simulink model "sm_car_testrig_susp_dwa_hp"  (R2025b)
settings: Solver=ode23t  StartTime=0.0  StopTime=1e-9  RelTol=1e-3  EnableMultiTasking=on
PostLoadFcn:
  | sm_car_load_vehicle_data(bdroot,'016');
undefined symbols (not defined in the file): Init, LAf, LAr, UAf, UAr, Vehicle, X, Y, Z
libraries: sm_lib x102, nesl_utility x67, Suspension_Utilities x8, Linkage_Arms x6, Linkage_DW_A x4, fl_lib x4, Linkage_Shock x2, Linkage_Uprights x2
(part 1 of 4)
Description:
  | Hardpoint Testrig for Double-Wishbone, Design A
  | 
  | Copyright 2018-2025 The MathWorks, Inc.
settings Model: Creator=smiller  LastModifiedBy=smiller
settings SolverCC: AlgebraicLoopSolver=TrustRegion
settings DataIOCC: LimitDataPoints=on  ReturnWorkspaceOutputs=off
settings OptimizationCC: ReuseModelBlockBuffer=off  LifeSpan=inf
settings DebuggingCC: UnconnectedInputMsg=warning  UnconnectedOutputMsg=warning  UnconnectedLineMsg=warning  AllowSymbolicDim=off  SFUnexpectedBacktrackingDiag=warning  SFNoUnconditionalDefaultTransitionDiag=warning  SFExecutionAtInitializationDiag=none  ArithmeticOperatorsInVariantConditions=warning
settings ModelReferenceCC: EnableRefExpFcnMdlSchedulingChecks=on
settings SFSimCC: SimUseLocalCustomCode=off  CustomCodeUndefinedFunction=UseInterfaceOnly
settings RTWCC: RTWUseLocalCustomCode=off  GPUComputeCapability=3.5  DLArmComputeVersion=19.05
settings CodeAppCC: StateflowObjectComments=on
settings GRTTargetCC: TargetLangStandard=C89/C90 (ANSI)
settings ConfigComp: CovMetricSettings=dw  CovSaveCumulativeToWorkspaceVar=on  CovSaveSingleToWorkspaceVar=on  CovExternalEMLEnable=off  CovSFcnEnable=off
settings SimscapeCC: SimscapeNominalValues="[{\"value\":\"10\",\"unit\":\"V\"},{\"value\":\"1\",\"unit\":\"A\"},{\"value\":\"10\",\"unit\":\"N*m\"},{\"value\":\"10\",\"unit\":\"bar\"},{\"value\":\"100\",\"unit\":\"kJ/kg\"},{\"value\":\"1\",\"unit\":\"kW\"},{\"value\":\"300\",\"unit\":\"K\"},{\"value\":\"100\",\"unit\":\"cm^3/s\"},{\"value\":\"1\",\"unit\":\"kN\"},{\"value\":\"1\",\"unit\":\"g/cm^3\"},{\"value\":\"1\",\"unit\":\"l\"},{\"value\":\"1\",\"unit\":\"cm^2\"},{\"value\":\"60\",\"unit\":\"Hz\"}]"  SimscapeLogType=all  SimscapeLogDataHistory=10000.0
settings ConfigurationSet: Description=SimMechanics 2G
settings ExplorerConfigSet: InternalSimMechanicsExplorerSettings="<ExplorerConfiguration><canonicalview>default</canonicalview><AnimationSetting><BasePlaybackSpeed>1.0</BasePlaybackSpeed><PlaybackSpeedFactor>1.0</PlaybackSpeedFactor></AnimationSetting><TilePanel><TileInfo><Tiles Columns=\"1\" Count=\"2\" Rows=\"2\"><Column Weight=\"1\"/><Row Weight=\"0.4725\"/><Row Weight=\"0.5275\"/><Tile Height=\"1\" Width=\"1\" X=\"0\" Y=\"0\"/><Tile Height=\"1\" Width=\"1\" X=\"0\" Y=\"1\"/></Tiles></TileInfo><SceneInfo><SceneViewer><BGColor><R>1</R><G>1</G><B>1</B></BGColor><Camera><DoPerspective>off</DoPerspective><Position><X>0.0507207717361932015</X><Y>0.00200032852270663059</Y><Z>1.76122408385226614</Z></Position><Center><X>0.0507207717361932015</X><Y>0.00200032852270663059</Y><Z>0.418399934818852515</Z></Center><Up><X>0.999884344159155392</X><Y>0.015208494515101291</Y><Z>0</Z></Up><ViewLimDist>1</ViewLimDist><YLim>0.36770677816381625</YLim><XLim>1.19032707650096015</XLim></Camera></SceneViewer><SceneViewer><BGColor><R>1</R><G>1</G><B>1</B></BGColor><Camera><DoPerspective>off</DoPerspective><Position><X>-1.166386773956821</X><Y>3.31266427622267656e-08</Y><Z>0.418399978770330305</Z></Position><Center><X>0.0499999423256101139</X><Y>3.31266427622267656e-08</Y><Z>0.418399978770330305</Z></Center><Up><X>0</X><Y>0</Y><Z>1</Z></Up><ViewLimDist>1</ViewLimDist><YLim>0.416223000884056116</YLim><XLim>1.20586269840369886</XLim></Camera></SceneViewer></SceneInfo></TilePanel><MechEditorPanel><Cameras/><GfxPanelCameraMap/><VideoCreator><PlaybackSpeedRatio>1.0</PlaybackSpeedRatio><FrameRate>30</FrameRate><VideoFormat>Motion JPEG AVI</VideoFormat><FrameSize>auto</FrameSize></VideoCreator></MechEditorPanel></ExplorerConfiguration>"

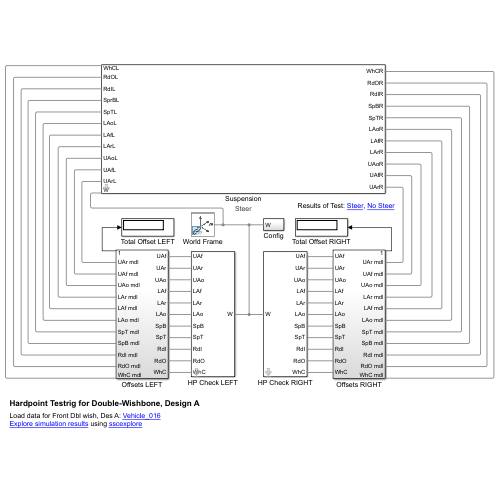
[thumbnail: Simulink's stored preview of the top-level diagram]
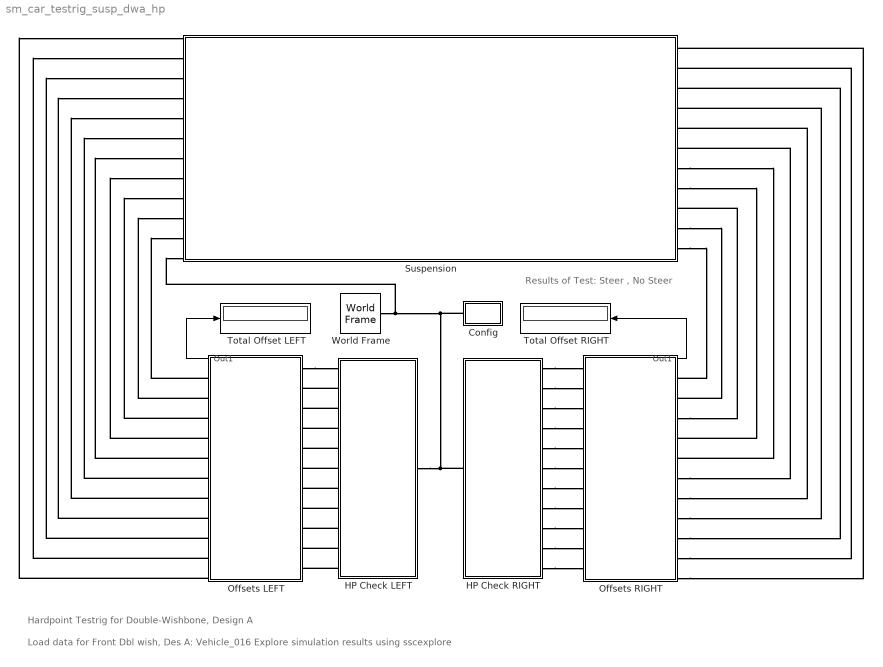
== system sm_car_testrig_susp_dwa_hp ==
  note: Results of Test: Steer , No Steer
  note: Hardpoint Testrig for Double-Wishbone, Design A
  note: Load data for Front Dbl wish, Des A: Vehicle_016
      | Explore simulation results using sscexplore
  Config : Subsystem
  HP Check LEFT : Subsystem  mask{Linkage=Vehicle.Chassis.SuspA1.Linkage, popup_leftRight=Left, rad_vis_sph=5e-2, clr_vis_sph=[0.4 0.4 1.0], opc_vis_sph=0.4, size_frm_vis=20, clr_frm_vis=[0.4 0.4 1.0], opc_frm_vis=0.5}
      mask prompts: Linkage "Linkage Parameters"; popup_leftRight "Left/Right"; rad_vis_sph "Sphere Radius (m)"; clr_vis_sph "Sphere Color [RGB]"; opc_vis_sph "Sphere Opacity (0-1)"; size_frm_vis "Frame Size (pixels)"; clr_frm_vis "Frame Color [RGB]"; opc_frm_vis "Frame Opacity (0-1)"
      mask init:
      | if(popup_leftRight==1)
      |     rhs_hp = [1 1 1];
      | elseif (popup_leftRight==2)
      |     rhs_hp = [1 -1 1];
      | end
      mask TypeOptions popup_leftRight: Left | Right
  HP Check RIGHT : Subsystem  mask{Linkage=Vehicle.Chassis.SuspA1.Linkage, popup_leftRight=Right, rad_vis_sph=5e-2, clr_vis_sph=[0.4 0.4 1.0], opc_vis_sph=0.4, size_frm_vis=20, clr_frm_vis=[0.4 0.4 1.0], opc_frm_vis=0.5}
      mask prompts: Linkage "Linkage Parameters"; popup_leftRight "Left/Right"; rad_vis_sph "Sphere Radius (m)"; clr_vis_sph "Sphere Color [RGB]"; opc_vis_sph "Sphere Opacity (0-1)"; size_frm_vis "Frame Size (pixels)"; clr_frm_vis "Frame Color [RGB]"; opc_frm_vis "Frame Opacity (0-1)"
      mask init:
      | if(popup_leftRight==1)
      |     rhs_hp = [1 1 1];
      | elseif (popup_leftRight==2)
      |     rhs_hp = [1 -1 1];
      | end
      mask TypeOptions popup_leftRight: Left | Right
  Offsets LEFT : Subsystem
  Offsets RIGHT : Subsystem
  Suspension : Subsystem  mask{popup_steer=Steer, Linkage=Vehicle.Chassis.SuspA1.Linkage}
      mask prompts: popup_steer "Steer (On/Off)"; Linkage "Linkage Parameters"
      mask init:
      | if (popup_steer == 1)
      |     set_param([gcb '/Track Rod LEFT'],'OverrideUsingVariant','Steer');
      |     set_param([gcb '/LA Upright LEFT'],'OverrideUsingVariant','Steer');
      |     set_param([gcb '/Track Rod RIGHT'],'OverrideUsingVariant','Steer');
      |     set_param([gcb '/LA Upright RIGHT'],'OverrideUsingVariant','Steer');
      | elseif (popup_steer == 2)
      |     set_param([gcb '/Track Rod LEFT'],'OverrideUsingVariant','No_Steer');
      |     set_param([gcb '/LA Upright LEFT'],'OverrideUsingVariant','No_Steer');
      |     set_param([gcb '/Track Rod RIGHT'],'OverrideUsingVariant','No_Steer');
      |     set_param([gcb '/LA Upright RIGHT'],'OverrideUsingVariant','No_Steer');
      | end
      settings: AttributesFormatString=%<popup_steer>
      mask TypeOptions popup_steer: Steer | No Steer
  Total Offset LEFT : Display
  Total Offset RIGHT : Display
  World Frame : sm_lib/Frames and Transforms/World Frame
  wires:
  Offsets LEFT/1(Out1) -> Total Offset LEFT/1
  Offsets RIGHT/1(Out1) -> Total Offset RIGHT/1
  connections:
  Offsets LEFT/LConn1 -- HP Check LEFT/RConn1
  HP Check LEFT/RConn2 -- Offsets LEFT/LConn2
  HP Check LEFT/RConn3 -- Offsets LEFT/LConn3
  HP Check LEFT/RConn4 -- Offsets LEFT/LConn4
  HP Check LEFT/RConn5 -- Offsets LEFT/LConn5
  HP Check LEFT/RConn6 -- Offsets LEFT/LConn6
  HP Check LEFT/RConn7 -- Offsets LEFT/LConn7
  HP Check LEFT/RConn8 -- Offsets LEFT/LConn8
  HP Check LEFT/RConn9 -- Offsets LEFT/LConn9
  HP Check LEFT/RConn10 -- Offsets LEFT/LConn10
  HP Check LEFT/RConn11 -- Offsets LEFT/LConn11
  HP Check RIGHT/RConn1 -- Offsets RIGHT/LConn1
  HP Check RIGHT/RConn2 -- Offsets RIGHT/LConn2
  HP Check RIGHT/RConn3 -- Offsets RIGHT/LConn3
  HP Check RIGHT/RConn4 -- Offsets RIGHT/LConn4
  HP Check RIGHT/RConn5 -- Offsets RIGHT/LConn5
  HP Check RIGHT/RConn6 -- Offsets RIGHT/LConn6
  HP Check RIGHT/RConn7 -- Offsets RIGHT/LConn7
  HP Check RIGHT/RConn8 -- Offsets RIGHT/LConn8
  HP Check RIGHT/RConn9 -- Offsets RIGHT/LConn9
  HP Check RIGHT/RConn10 -- Offsets RIGHT/LConn10
  HP Check RIGHT/RConn11 -- Offsets RIGHT/LConn11
  World Frame/RConn1 -- HP Check RIGHT/LConn1 -- HP Check LEFT/LConn1 -- Config/LConn1 -- Suspension/LConn12
  Offsets LEFT/RConn1 -- Suspension/LConn11
  Suspension/RConn11 -- Offsets RIGHT/RConn1
  Offsets LEFT/RConn2 -- Suspension/LConn10
  Suspension/RConn10 -- Offsets RIGHT/RConn2
  Offsets LEFT/RConn3 -- Suspension/LConn9
  Offsets RIGHT/RConn3 -- Suspension/RConn9
  Offsets LEFT/RConn4 -- Suspension/LConn8
  Suspension/RConn8 -- Offsets RIGHT/RConn4
  Offsets LEFT/RConn5 -- Suspension/LConn7
  Suspension/RConn7 -- Offsets RIGHT/RConn5
  Offsets LEFT/RConn6 -- Suspension/LConn6
  Offsets RIGHT/RConn6 -- Suspension/RConn6
  Offsets LEFT/RConn7 -- Suspension/LConn5
  Offsets RIGHT/RConn7 -- Suspension/RConn5
  Offsets LEFT/RConn8 -- Suspension/LConn4
  Offsets RIGHT/RConn8 -- Suspension/RConn4
  Offsets LEFT/RConn9 -- Suspension/LConn3
  Offsets RIGHT/RConn9 -- Suspension/RConn3
  Offsets LEFT/RConn10 -- Suspension/LConn2
  Offsets RIGHT/RConn10 -- Suspension/RConn2
  Offsets LEFT/RConn11 -- Suspension/LConn1
  Offsets RIGHT/RConn11 -- Suspension/RConn1

== system sm_car_testrig_susp_dwa_hp/Config ==
  Mechanism Configuration : sm_lib/Utilities/Mechanism Configuration  UniformGravity=Constant  GravityVector=[0 0 -9.80665]  GravityVectorUnits=m/s^2  LinearizationDelta=0.001  JointModeTransitionNonlinearIterations=2
  Solver Configuration : nesl_utility/Solver Configuration  PhysicalDomain=network_engine_domain  SubClassName=solver  LeftPortType=input  RightPortType=generic  Tones=[]  Harmonics=[]  SimulateNoise=off  Profile=off  UseLocalSampling=off  EnableSwitchedLinearOptims=on  FrequencyDomain=off  UseCCode=off  RelTol=0.001  AbsTol=1e-06  MinStep=1e-09  ToWorkspace=off  RevertToSquareIcSolve=off  NumHomotopyIterations=100  PhasorMode=off  PhasorModeNumHarmonics=1  ConsistencySolver=NEWTON_FTOL  IndexReductionMethod=DerivativeReplacement  DoDC=off  ResidualTolerance=1e-09  ConsistencyTolSource=GLOBAL  ConsistencyAbsTol=0.001  ConsistencyRelTol=0.001  ConsistencyTolFactor=0.001  UseLocalSolver=off  LocalSolverChoice=NE_BACKWARD_EULER_ADVANCER  ResolveIndetEquations=on  FunctionEvalNumThread=1  LocalSolverSampleTime=0.001  DoFixedCost=off  MaxNonlinIter=3  MaxModeIter=2  ComputeImpulses=off  ImpulseIterations=2  LinearAlgebra=Sparse  LinearAlgebraNumThread=0  EquationFormulation=NE_TIME_EF  DelaysMemoryBudget=1024  AutomaticFiltering=on  FilteringTimeConstant=0.001  PartitionStorageMethod=AS_NEEDED  PartitionMemoryBudget=1024  PartitionMethod=FAST  MultibodyUseLocalSolver=off  MultibodyLocalSolverChoice=ODE1  MultibodyLocalSolverSampleTime=0.001
  W : PMIOPort  Side=Left
  connections:
  Mechanism Configuration/RConn1 -- Solver Configuration/RConn1 -- W/RConn1

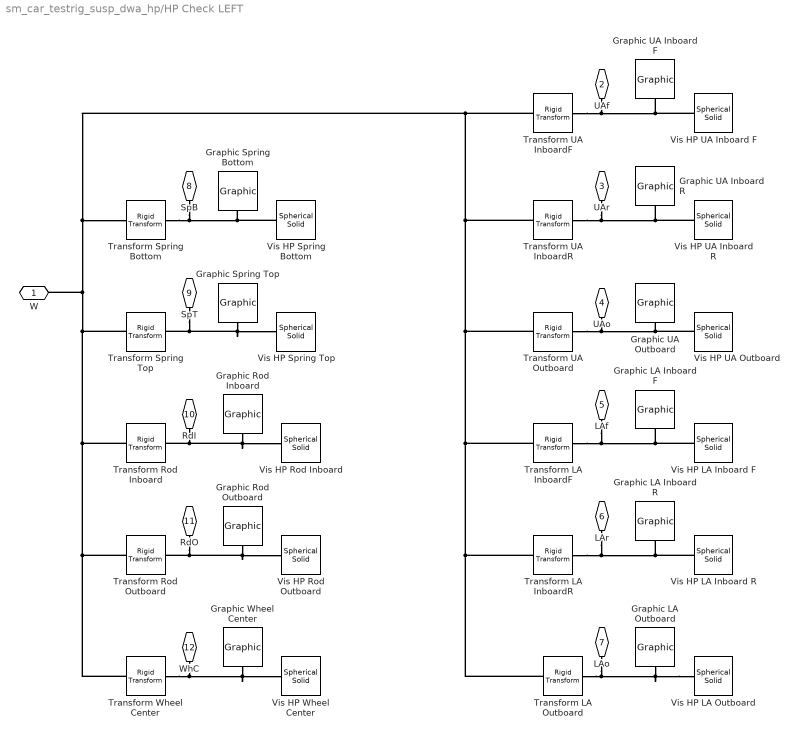
== system sm_car_testrig_susp_dwa_hp/HP Check LEFT ==
  Graphic LA Inboard F : sm_lib/Body Elements/Graphic  GraphicType=Marker  MarkerShape=Frame  MarkerSize=size_frm_vis  GraphicVisPropType=SimpleVisualProperties  GraphicDiffuseColor=clr_frm_vis  GraphicOpacity=opc_frm_vis  GraphicSpecularColor=[0.5 0.5 0.5 1.0]  GraphicAmbientColor=[0.15 0.15 0.15 1.0]  GraphicEmissiveColor=[0.0 0.0 0.0 1.0]  GraphicShininess=75
  Graphic LA Inboard R : sm_lib/Body Elements/Graphic  GraphicType=Marker  MarkerShape=Frame  MarkerSize=size_frm_vis  GraphicVisPropType=SimpleVisualProperties  GraphicDiffuseColor=clr_frm_vis  GraphicOpacity=opc_frm_vis  GraphicSpecularColor=[0.5 0.5 0.5 1.0]  GraphicAmbientColor=[0.15 0.15 0.15 1.0]  GraphicEmissiveColor=[0.0 0.0 0.0 1.0]  GraphicShininess=75
  Graphic LA Outboard : sm_lib/Body Elements/Graphic  GraphicType=Marker  MarkerShape=Frame  MarkerSize=size_frm_vis  GraphicVisPropType=SimpleVisualProperties  GraphicDiffuseColor=clr_frm_vis  GraphicOpacity=opc_frm_vis  GraphicSpecularColor=[0.5 0.5 0.5 1.0]  GraphicAmbientColor=[0.15 0.15 0.15 1.0]  GraphicEmissiveColor=[0.0 0.0 0.0 1.0]  GraphicShininess=75
  Graphic Rod Inboard : sm_lib/Body Elements/Graphic  GraphicType=Marker  MarkerShape=Frame  MarkerSize=size_frm_vis  GraphicVisPropType=SimpleVisualProperties  GraphicDiffuseColor=clr_frm_vis  GraphicOpacity=opc_frm_vis  GraphicSpecularColor=[0.5 0.5 0.5 1.0]  GraphicAmbientColor=[0.15 0.15 0.15 1.0]  GraphicEmissiveColor=[0.0 0.0 0.0 1.0]  GraphicShininess=75
  Graphic Rod Outboard : sm_lib/Body Elements/Graphic  GraphicType=Marker  MarkerShape=Frame  MarkerSize=size_frm_vis  GraphicVisPropType=SimpleVisualProperties  GraphicDiffuseColor=clr_frm_vis  GraphicOpacity=opc_frm_vis  GraphicSpecularColor=[0.5 0.5 0.5 1.0]  GraphicAmbientColor=[0.15 0.15 0.15 1.0]  GraphicEmissiveColor=[0.0 0.0 0.0 1.0]  GraphicShininess=75
  Graphic Spring Bottom : sm_lib/Body Elements/Graphic  GraphicType=Marker  MarkerShape=Frame  MarkerSize=size_frm_vis  GraphicVisPropType=SimpleVisualProperties  GraphicDiffuseColor=clr_frm_vis  GraphicOpacity=opc_frm_vis  GraphicSpecularColor=[0.5 0.5 0.5 1.0]  GraphicAmbientColor=[0.15 0.15 0.15 1.0]  GraphicEmissiveColor=[0.0 0.0 0.0 1.0]  GraphicShininess=75
  Graphic Spring Top : sm_lib/Body Elements/Graphic  GraphicType=Marker  MarkerShape=Frame  MarkerSize=size_frm_vis  GraphicVisPropType=SimpleVisualProperties  GraphicDiffuseColor=clr_frm_vis  GraphicOpacity=opc_frm_vis  GraphicSpecularColor=[0.5 0.5 0.5 1.0]  GraphicAmbientColor=[0.15 0.15 0.15 1.0]  GraphicEmissiveColor=[0.0 0.0 0.0 1.0]  GraphicShininess=75
  Graphic UA Inboard F : sm_lib/Body Elements/Graphic  GraphicType=Marker  MarkerShape=Frame  MarkerSize=size_frm_vis  GraphicVisPropType=SimpleVisualProperties  GraphicDiffuseColor=clr_frm_vis  GraphicOpacity=opc_frm_vis  GraphicSpecularColor=[0.5 0.5 0.5 1.0]  GraphicAmbientColor=[0.15 0.15 0.15 1.0]  GraphicEmissiveColor=[0.0 0.0 0.0 1.0]  GraphicShininess=75
  Graphic UA Inboard R : sm_lib/Body Elements/Graphic  GraphicType=Marker  MarkerShape=Frame  MarkerSize=size_frm_vis  GraphicVisPropType=SimpleVisualProperties  GraphicDiffuseColor=clr_frm_vis  GraphicOpacity=opc_frm_vis  GraphicSpecularColor=[0.5 0.5 0.5 1.0]  GraphicAmbientColor=[0.15 0.15 0.15 1.0]  GraphicEmissiveColor=[0.0 0.0 0.0 1.0]  GraphicShininess=75
  Graphic UA Outboard : sm_lib/Body Elements/Graphic  GraphicType=Marker  MarkerShape=Frame  MarkerSize=size_frm_vis  GraphicVisPropType=SimpleVisualProperties  GraphicDiffuseColor=clr_frm_vis  GraphicOpacity=opc_frm_vis  GraphicSpecularColor=[0.5 0.5 0.5 1.0]  GraphicAmbientColor=[0.15 0.15 0.15 1.0]  GraphicEmissiveColor=[0.0 0.0 0.0 1.0]  GraphicShininess=75
  Graphic Wheel Center : sm_lib/Body Elements/Graphic  GraphicType=Marker  MarkerShape=Frame  MarkerSize=size_frm_vis  GraphicVisPropType=SimpleVisualProperties  GraphicDiffuseColor=clr_frm_vis  GraphicOpacity=opc_frm_vis  GraphicSpecularColor=[0.5 0.5 0.5 1.0]  GraphicAmbientColor=[0.15 0.15 0.15 1.0]  GraphicEmissiveColor=[0.0 0.0 0.0 1.0]  GraphicShininess=75
  Transform LA InboardF : sm_lib/Frames and Transforms/Rigid Transform  RotationMethod=None  FollAlignAxisA=+X  BaseAlignAxisA=+Y  FollAlignAxisB=+Y  BaseAlignAxisB=+Z  RotationStandardAxis=+Z  RotationAngle=0.0  RotationAngleUnits=deg  RotationArbitraryAxis=[0 0 1]  RotationSequenceAxes=FollowerAxes  RotationSequence=XYX  RotationSequenceAngles=[0 0 0]  RotationSequenceAnglesUnits=deg  RotationMatrix=[1 0 0; 0 1 0; 0 0 1]  Quaternion=[1 0 0 0]  TranslationMethod=Cartesian  TranslationCartesianOffset=Linkage.LowerWishbone.sInboardF.Value.*rhs_hp  TranslationCartesianOffsetUnits=m  TranslationStandardAxis=+Z  TranslationStandardOffset=0  TranslationStandardOffsetUnits=m  TranslationROffset=0  TranslationROffsetUnits=m  TranslationThetaOffset=0  TranslationThetaOffsetUnits=deg  TranslationZOffset=0  TranslationZOffsetUnits=m
      settings: AttributesFormatString=%<TranslationCartesianOffset>
  Transform LA InboardR : sm_lib/Frames and Transforms/Rigid Transform  RotationMethod=None  FollAlignAxisA=+X  BaseAlignAxisA=+Y  FollAlignAxisB=+Y  BaseAlignAxisB=+Z  RotationStandardAxis=+Z  RotationAngle=0.0  RotationAngleUnits=deg  RotationArbitraryAxis=[0 0 1]  RotationSequenceAxes=FollowerAxes  RotationSequence=XYX  RotationSequenceAngles=[0 0 0]  RotationSequenceAnglesUnits=deg  RotationMatrix=[1 0 0; 0 1 0; 0 0 1]  Quaternion=[1 0 0 0]  TranslationMethod=Cartesian  TranslationCartesianOffset=Linkage.LowerWishbone.sInboardR.Value.*rhs_hp  TranslationCartesianOffsetUnits=m  TranslationStandardAxis=+Z  TranslationStandardOffset=0  TranslationStandardOffsetUnits=m  TranslationROffset=0  TranslationROffsetUnits=m  TranslationThetaOffset=0  TranslationThetaOffsetUnits=deg  TranslationZOffset=0  TranslationZOffsetUnits=m
      settings: AttributesFormatString=%<TranslationCartesianOffset>
  Transform LA Outboard : sm_lib/Frames and Transforms/Rigid Transform  RotationMethod=None  FollAlignAxisA=+X  BaseAlignAxisA=+Y  FollAlignAxisB=+Y  BaseAlignAxisB=+Z  RotationStandardAxis=+Z  RotationAngle=0.0  RotationAngleUnits=deg  RotationArbitraryAxis=[0 0 1]  RotationSequenceAxes=FollowerAxes  RotationSequence=XYX  RotationSequenceAngles=[0 0 0]  RotationSequenceAnglesUnits=deg  RotationMatrix=[1 0 0; 0 1 0; 0 0 1]  Quaternion=[1 0 0 0]  TranslationMethod=Cartesian  TranslationCartesianOffset=Linkage.LowerWishbone.sOutboard.Value.*rhs_hp  TranslationCartesianOffsetUnits=m  TranslationStandardAxis=+Z  TranslationStandardOffset=0  TranslationStandardOffsetUnits=m  TranslationROffset=0  TranslationROffsetUnits=m  TranslationThetaOffset=0  TranslationThetaOffsetUnits=deg  TranslationZOffset=0  TranslationZOffsetUnits=m
      settings: AttributesFormatString=%<TranslationCartesianOffset>
  Transform Rod Inboard : sm_lib/Frames and Transforms/Rigid Transform  RotationMethod=None  FollAlignAxisA=+X  BaseAlignAxisA=+Y  FollAlignAxisB=+Y  BaseAlignAxisB=+Z  RotationStandardAxis=+Z  RotationAngle=0.0  RotationAngleUnits=deg  RotationArbitraryAxis=[0 0 1]  RotationSequenceAxes=FollowerAxes  RotationSequence=XYX  RotationSequenceAngles=[0 0 0]  RotationSequenceAnglesUnits=deg  RotationMatrix=[1 0 0; 0 1 0; 0 0 1]  Quaternion=[1 0 0 0]  TranslationMethod=Cartesian  TranslationCartesianOffset=Linkage.TrackRod.sInboard.Value.*rhs_hp  TranslationCartesianOffsetUnits=m  TranslationStandardAxis=+Z  TranslationStandardOffset=0  TranslationStandardOffsetUnits=m  TranslationROffset=0  TranslationROffsetUnits=m  TranslationThetaOffset=0  TranslationThetaOffsetUnits=deg  TranslationZOffset=0  TranslationZOffsetUnits=m
      settings: AttributesFormatString=%<TranslationCartesianOffset>
  Transform Rod Outboard : sm_lib/Frames and Transforms/Rigid Transform  RotationMethod=None  FollAlignAxisA=+X  BaseAlignAxisA=+Y  FollAlignAxisB=+Y  BaseAlignAxisB=+Z  RotationStandardAxis=+Z  RotationAngle=0.0  RotationAngleUnits=deg  RotationArbitraryAxis=[0 0 1]  RotationSequenceAxes=FollowerAxes  RotationSequence=XYX  RotationSequenceAngles=[0 0 0]  RotationSequenceAnglesUnits=deg  RotationMatrix=[1 0 0; 0 1 0; 0 0 1]  Quaternion=[1 0 0 0]  TranslationMethod=Cartesian  TranslationCartesianOffset=Linkage.TrackRod.sOutboard.Value.*rhs_hp  TranslationCartesianOffsetUnits=m  TranslationStandardAxis=+Z  TranslationStandardOffset=0  TranslationStandardOffsetUnits=m  TranslationROffset=0  TranslationROffsetUnits=m  TranslationThetaOffset=0  TranslationThetaOffsetUnits=deg  TranslationZOffset=0  TranslationZOffsetUnits=m
      settings: AttributesFormatString=%<TranslationCartesianOffset>
  Transform Spring Bottom : sm_lib/Frames and Transforms/Rigid Transform  RotationMethod=None  FollAlignAxisA=+X  BaseAlignAxisA=+Y  FollAlignAxisB=+Y  BaseAlignAxisB=+Z  RotationStandardAxis=+Z  RotationAngle=0.0  RotationAngleUnits=deg  RotationArbitraryAxis=[0 0 1]  RotationSequenceAxes=FollowerAxes  RotationSequence=XYX  RotationSequenceAngles=[0 0 0]  RotationSequenceAnglesUnits=deg  RotationMatrix=[1 0 0; 0 1 0; 0 0 1]  Quaternion=[1 0 0 0]  TranslationMethod=Cartesian  TranslationCartesianOffset=Linkage.Shock.sBottom.Value.*rhs_hp  TranslationCartesianOffsetUnits=m  TranslationStandardAxis=+Z  TranslationStandardOffset=0  TranslationStandardOffsetUnits=m  TranslationROffset=0  TranslationROffsetUnits=m  TranslationThetaOffset=0  TranslationThetaOffsetUnits=deg  TranslationZOffset=0  TranslationZOffsetUnits=m
      settings: AttributesFormatString=%<TranslationCartesianOffset>
  Transform Spring Top : sm_lib/Frames and Transforms/Rigid Transform  RotationMethod=None  FollAlignAxisA=+X  BaseAlignAxisA=+Y  FollAlignAxisB=+Y  BaseAlignAxisB=+Z  RotationStandardAxis=+Z  RotationAngle=0.0  RotationAngleUnits=deg  RotationArbitraryAxis=[0 0 1]  RotationSequenceAxes=FollowerAxes  RotationSequence=XYX  RotationSequenceAngles=[0 0 0]  RotationSequenceAnglesUnits=deg  RotationMatrix=[1 0 0; 0 1 0; 0 0 1]  Quaternion=[1 0 0 0]  TranslationMethod=Cartesian  TranslationCartesianOffset=Linkage.Shock.sTop.Value.*rhs_hp  TranslationCartesianOffsetUnits=m  TranslationStandardAxis=+Z  TranslationStandardOffset=0  TranslationStandardOffsetUnits=m  TranslationROffset=0  TranslationROffsetUnits=m  TranslationThetaOffset=0  TranslationThetaOffsetUnits=deg  TranslationZOffset=0  TranslationZOffsetUnits=m
      settings: AttributesFormatString=%<TranslationCartesianOffset>
  Transform UA InboardF : sm_lib/Frames and Transforms/Rigid Transform  RotationMethod=None  FollAlignAxisA=+X  BaseAlignAxisA=+Y  FollAlignAxisB=+Y  BaseAlignAxisB=+Z  RotationStandardAxis=+Z  RotationAngle=0.0  RotationAngleUnits=deg  RotationArbitraryAxis=[0 0 1]  RotationSequenceAxes=FollowerAxes  RotationSequence=XYX  RotationSequenceAngles=[0 0 0]  RotationSequenceAnglesUnits=deg  RotationMatrix=[1 0 0; 0 1 0; 0 0 1]  Quaternion=[1 0 0 0]  TranslationMethod=Cartesian  TranslationCartesianOffset=Linkage.UpperWishbone.sInboardF.Value.*rhs_hp  TranslationCartesianOffsetUnits=m  TranslationStandardAxis=+Z  TranslationStandardOffset=0  TranslationStandardOffsetUnits=m  TranslationROffset=0  TranslationROffsetUnits=m  TranslationThetaOffset=0  TranslationThetaOffsetUnits=deg  TranslationZOffset=0  TranslationZOffsetUnits=m
      settings: AttributesFormatString=%<TranslationCartesianOffset>
  Transform UA InboardR : sm_lib/Frames and Transforms/Rigid Transform  RotationMethod=None  FollAlignAxisA=+X  BaseAlignAxisA=+Y  FollAlignAxisB=+Y  BaseAlignAxisB=+Z  RotationStandardAxis=+Z  RotationAngle=0.0  RotationAngleUnits=deg  RotationArbitraryAxis=[0 0 1]  RotationSequenceAxes=FollowerAxes  RotationSequence=XYX  RotationSequenceAngles=[0 0 0]  RotationSequenceAnglesUnits=deg  RotationMatrix=[1 0 0; 0 1 0; 0 0 1]  Quaternion=[1 0 0 0]  TranslationMethod=Cartesian  TranslationCartesianOffset=Linkage.UpperWishbone.sInboardR.Value.*rhs_hp  TranslationCartesianOffsetUnits=m  TranslationStandardAxis=+Z  TranslationStandardOffset=0  TranslationStandardOffsetUnits=m  TranslationROffset=0  TranslationROffsetUnits=m  TranslationThetaOffset=0  TranslationThetaOffsetUnits=deg  TranslationZOffset=0  TranslationZOffsetUnits=m
      settings: AttributesFormatString=%<TranslationCartesianOffset>
  Transform UA Outboard : sm_lib/Frames and Transforms/Rigid Transform  RotationMethod=None  FollAlignAxisA=+X  BaseAlignAxisA=+Y  FollAlignAxisB=+Y  BaseAlignAxisB=+Z  RotationStandardAxis=+Z  RotationAngle=0.0  RotationAngleUnits=deg  RotationArbitraryAxis=[0 0 1]  RotationSequenceAxes=FollowerAxes  RotationSequence=XYX  RotationSequenceAngles=[0 0 0]  RotationSequenceAnglesUnits=deg  RotationMatrix=[1 0 0; 0 1 0; 0 0 1]  Quaternion=[1 0 0 0]  TranslationMethod=Cartesian  TranslationCartesianOffset=Linkage.UpperWishbone.sOutboard.Value.*rhs_hp  TranslationCartesianOffsetUnits=m  TranslationStandardAxis=+Z  TranslationStandardOffset=0  TranslationStandardOffsetUnits=m  TranslationROffset=0  TranslationROffsetUnits=m  TranslationThetaOffset=0  TranslationThetaOffsetUnits=deg  TranslationZOffset=0  TranslationZOffsetUnits=m
      settings: AttributesFormatString=%<TranslationCartesianOffset>
  Transform Wheel Center : sm_lib/Frames and Transforms/Rigid Transform  RotationMethod=None  FollAlignAxisA=+X  BaseAlignAxisA=+Y  FollAlignAxisB=+Y  BaseAlignAxisB=+Z  RotationStandardAxis=+Z  RotationAngle=0.0  RotationAngleUnits=deg  RotationArbitraryAxis=[0 0 1]  RotationSequenceAxes=FollowerAxes  RotationSequence=XYX  RotationSequenceAngles=[0 0 0]  RotationSequenceAnglesUnits=deg  RotationMatrix=[1 0 0; 0 1 0; 0 0 1]  Quaternion=[1 0 0 0]  TranslationMethod=Cartesian  TranslationCartesianOffset=Linkage.Upright.sWheelCentre.Value.*rhs_hp  TranslationCartesianOffsetUnits=m  TranslationStandardAxis=+Z  TranslationStandardOffset=0  TranslationStandardOffsetUnits=m  TranslationROffset=0  TranslationROffsetUnits=m  TranslationThetaOffset=0  TranslationThetaOffsetUnits=deg  TranslationZOffset=0  TranslationZOffsetUnits=m
      settings: AttributesFormatString=%<TranslationCartesianOffset>
  Vis HP LA Inboard F : sm_lib/Body Elements/Spherical Solid  SphereRadius=rad_vis_sph  SphereRadiusUnits=m  ExportEntireGeometry=off  InertiaType=CalculateFromGeometry  BasedOnType=Density  Density=1000  DensityUnits=kg/m^3  Mass=1  MassUnits=kg  CenterOfMass=[0 0 0]  CenterOfMassUnits=m  MomentsOfInertia=[1 1 1]  MomentsOfInertiaUnits=kg*m^2  ProductsOfInertia=[0 0 0]  ProductsOfInertiaUnits=kg*m^2  GraphicType=FromGeometry  MarkerShape=Sphere  MarkerSize=10  GraphicVisPropType=SimpleVisualProperties  GraphicDiffuseColor=clr_vis_sph  GraphicOpacity=opc_vis_sph  GraphicSpecularColor=[0.5 0.5 0.5 1.0]  GraphicAmbientColor=[0.15 0.15 0.15 1.0]  GraphicEmissiveColor=[0.0 0.0 0.0 1.0]  GraphicShininess=75  DoExposeReferenceFrame=on  SerializedFrames=<Frames/>
  Vis HP LA Inboard R : sm_lib/Body Elements/Spherical Solid  SphereRadius=rad_vis_sph  SphereRadiusUnits=m  ExportEntireGeometry=off  InertiaType=CalculateFromGeometry  BasedOnType=Density  Density=1000  DensityUnits=kg/m^3  Mass=1  MassUnits=kg  CenterOfMass=[0 0 0]  CenterOfMassUnits=m  MomentsOfInertia=[1 1 1]  MomentsOfInertiaUnits=kg*m^2  ProductsOfInertia=[0 0 0]  ProductsOfInertiaUnits=kg*m^2  GraphicType=FromGeometry  MarkerShape=Sphere  MarkerSize=10  GraphicVisPropType=SimpleVisualProperties  GraphicDiffuseColor=clr_vis_sph  GraphicOpacity=opc_vis_sph  GraphicSpecularColor=[0.5 0.5 0.5 1.0]  GraphicAmbientColor=[0.15 0.15 0.15 1.0]  GraphicEmissiveColor=[0.0 0.0 0.0 1.0]  GraphicShininess=75  DoExposeReferenceFrame=on  SerializedFrames=<Frames/>
  Vis HP LA Outboard : sm_lib/Body Elements/Spherical Solid  SphereRadius=rad_vis_sph  SphereRadiusUnits=m  ExportEntireGeometry=off  InertiaType=CalculateFromGeometry  BasedOnType=Density  Density=1000  DensityUnits=kg/m^3  Mass=1  MassUnits=kg  CenterOfMass=[0 0 0]  CenterOfMassUnits=m  MomentsOfInertia=[1 1 1]  MomentsOfInertiaUnits=kg*m^2  ProductsOfInertia=[0 0 0]  ProductsOfInertiaUnits=kg*m^2  GraphicType=FromGeometry  MarkerShape=Sphere  MarkerSize=10  GraphicVisPropType=SimpleVisualProperties  GraphicDiffuseColor=clr_vis_sph  GraphicOpacity=opc_vis_sph  GraphicSpecularColor=[0.5 0.5 0.5 1.0]  GraphicAmbientColor=[0.15 0.15 0.15 1.0]  GraphicEmissiveColor=[0.0 0.0 0.0 1.0]  GraphicShininess=75  DoExposeReferenceFrame=on  SerializedFrames=<Frames/>
  Vis HP Rod Inboard : sm_lib/Body Elements/Spherical Solid  SphereRadius=rad_vis_sph  SphereRadiusUnits=m  ExportEntireGeometry=off  InertiaType=CalculateFromGeometry  BasedOnType=Density  Density=1000  DensityUnits=kg/m^3  Mass=1  MassUnits=kg  CenterOfMass=[0 0 0]  CenterOfMassUnits=m  MomentsOfInertia=[1 1 1]  MomentsOfInertiaUnits=kg*m^2  ProductsOfInertia=[0 0 0]  ProductsOfInertiaUnits=kg*m^2  GraphicType=FromGeometry  MarkerShape=Sphere  MarkerSize=10  GraphicVisPropType=SimpleVisualProperties  GraphicDiffuseColor=clr_vis_sph  GraphicOpacity=opc_vis_sph  GraphicSpecularColor=[0.5 0.5 0.5 1.0]  GraphicAmbientColor=[0.15 0.15 0.15 1.0]  GraphicEmissiveColor=[0.0 0.0 0.0 1.0]  GraphicShininess=75  DoExposeReferenceFrame=on  SerializedFrames=<Frames/>
  Vis HP Rod Outboard : sm_lib/Body Elements/Spherical Solid  SphereRadius=rad_vis_sph  SphereRadiusUnits=m  ExportEntireGeometry=off  InertiaType=CalculateFromGeometry  BasedOnType=Density  Density=1000  DensityUnits=kg/m^3  Mass=1  MassUnits=kg  CenterOfMass=[0 0 0]  CenterOfMassUnits=m  MomentsOfInertia=[1 1 1]  MomentsOfInertiaUnits=kg*m^2  ProductsOfInertia=[0 0 0]  ProductsOfInertiaUnits=kg*m^2  GraphicType=FromGeometry  MarkerShape=Sphere  MarkerSize=10  GraphicVisPropType=SimpleVisualProperties  GraphicDiffuseColor=clr_vis_sph  GraphicOpacity=opc_vis_sph  GraphicSpecularColor=[0.5 0.5 0.5 1.0]  GraphicAmbientColor=[0.15 0.15 0.15 1.0]  GraphicEmissiveColor=[0.0 0.0 0.0 1.0]  GraphicShininess=75  DoExposeReferenceFrame=on  SerializedFrames=<Frames/>
  Vis HP Spring Bottom : sm_lib/Body Elements/Spherical Solid  SphereRadius=rad_vis_sph  SphereRadiusUnits=m  ExportEntireGeometry=off  InertiaType=CalculateFromGeometry  BasedOnType=Density  Density=1000  DensityUnits=kg/m^3  Mass=1  MassUnits=kg  CenterOfMass=[0 0 0]  CenterOfMassUnits=m  MomentsOfInertia=[1 1 1]  MomentsOfInertiaUnits=kg*m^2  ProductsOfInertia=[0 0 0]  ProductsOfInertiaUnits=kg*m^2  GraphicType=FromGeometry  MarkerShape=Sphere  MarkerSize=10  GraphicVisPropType=SimpleVisualProperties  GraphicDiffuseColor=clr_vis_sph  GraphicOpacity=opc_vis_sph  GraphicSpecularColor=[0.5 0.5 0.5 1.0]  GraphicAmbientColor=[0.15 0.15 0.15 1.0]  GraphicEmissiveColor=[0.0 0.0 0.0 1.0]  GraphicShininess=75  DoExposeReferenceFrame=on  SerializedFrames=<Frames/>
  Vis HP Spring Top : sm_lib/Body Elements/Spherical Solid  SphereRadius=rad_vis_sph  SphereRadiusUnits=m  ExportEntireGeometry=off  InertiaType=CalculateFromGeometry  BasedOnType=Density  Density=1000  DensityUnits=kg/m^3  Mass=1  MassUnits=kg  CenterOfMass=[0 0 0]  CenterOfMassUnits=m  MomentsOfInertia=[1 1 1]  MomentsOfInertiaUnits=kg*m^2  ProductsOfInertia=[0 0 0]  ProductsOfInertiaUnits=kg*m^2  GraphicType=FromGeometry  MarkerShape=Sphere  MarkerSize=10  GraphicVisPropType=SimpleVisualProperties  GraphicDiffuseColor=clr_vis_sph  GraphicOpacity=opc_vis_sph  GraphicSpecularColor=[0.5 0.5 0.5 1.0]  GraphicAmbientColor=[0.15 0.15 0.15 1.0]  GraphicEmissiveColor=[0.0 0.0 0.0 1.0]  GraphicShininess=75  DoExposeReferenceFrame=on  SerializedFrames=<Frames/>
  Vis HP UA Inboard F : sm_lib/Body Elements/Spherical Solid  SphereRadius=rad_vis_sph  SphereRadiusUnits=m  ExportEntireGeometry=off  InertiaType=CalculateFromGeometry  BasedOnType=Density  Density=1000  DensityUnits=kg/m^3  Mass=1  MassUnits=kg  CenterOfMass=[0 0 0]  CenterOfMassUnits=m  MomentsOfInertia=[1 1 1]  MomentsOfInertiaUnits=kg*m^2  ProductsOfInertia=[0 0 0]  ProductsOfInertiaUnits=kg*m^2  GraphicType=FromGeometry  MarkerShape=Sphere  MarkerSize=10  GraphicVisPropType=SimpleVisualProperties  GraphicDiffuseColor=clr_vis_sph  GraphicOpacity=opc_vis_sph  GraphicSpecularColor=[0.5 0.5 0.5 1.0]  GraphicAmbientColor=[0.15 0.15 0.15 1.0]  GraphicEmissiveColor=[0.0 0.0 0.0 1.0]  GraphicShininess=75  DoExposeReferenceFrame=on  SerializedFrames=<Frames/>
  Vis HP UA Inboard R : sm_lib/Body Elements/Spherical Solid  SphereRadius=rad_vis_sph  SphereRadiusUnits=m  ExportEntireGeometry=off  InertiaType=CalculateFromGeometry  BasedOnType=Density  Density=1000  DensityUnits=kg/m^3  Mass=1  MassUnits=kg  CenterOfMass=[0 0 0]  CenterOfMassUnits=m  MomentsOfInertia=[1 1 1]  MomentsOfInertiaUnits=kg*m^2  ProductsOfInertia=[0 0 0]  ProductsOfInertiaUnits=kg*m^2  GraphicType=FromGeometry  MarkerShape=Sphere  MarkerSize=10  GraphicVisPropType=SimpleVisualProperties  GraphicDiffuseColor=clr_vis_sph  GraphicOpacity=opc_vis_sph  GraphicSpecularColor=[0.5 0.5 0.5 1.0]  GraphicAmbientColor=[0.15 0.15 0.15 1.0]  GraphicEmissiveColor=[0.0 0.0 0.0 1.0]  GraphicShininess=75  DoExposeReferenceFrame=on  SerializedFrames=<Frames/>
  Vis HP UA Outboard : sm_lib/Body Elements/Spherical Solid  SphereRadius=rad_vis_sph  SphereRadiusUnits=m  ExportEntireGeometry=off  InertiaType=CalculateFromGeometry  BasedOnType=Density  Density=1000  DensityUnits=kg/m^3  Mass=1  MassUnits=kg  CenterOfMass=[0 0 0]  CenterOfMassUnits=m  MomentsOfInertia=[1 1 1]  MomentsOfInertiaUnits=kg*m^2  ProductsOfInertia=[0 0 0]  ProductsOfInertiaUnits=kg*m^2  GraphicType=FromGeometry  MarkerShape=Sphere  MarkerSize=10  GraphicVisPropType=SimpleVisualProperties  GraphicDiffuseColor=clr_vis_sph  GraphicOpacity=opc_vis_sph  GraphicSpecularColor=[0.5 0.5 0.5 1.0]  GraphicAmbientColor=[0.15 0.15 0.15 1.0]  GraphicEmissiveColor=[0.0 0.0 0.0 1.0]  GraphicShininess=75  DoExposeReferenceFrame=on  SerializedFrames=<Frames/>
  Vis HP Wheel Center : sm_lib/Body Elements/Spherical Solid  SphereRadius=rad_vis_sph  SphereRadiusUnits=m  ExportEntireGeometry=off  InertiaType=CalculateFromGeometry  BasedOnType=Density  Density=1000  DensityUnits=kg/m^3  Mass=1  MassUnits=kg  CenterOfMass=[0 0 0]  CenterOfMassUnits=m  MomentsOfInertia=[1 1 1]  MomentsOfInertiaUnits=kg*m^2  ProductsOfInertia=[0 0 0]  ProductsOfInertiaUnits=kg*m^2  GraphicType=FromGeometry  MarkerShape=Sphere  MarkerSize=10  GraphicVisPropType=SimpleVisualProperties  GraphicDiffuseColor=clr_vis_sph  GraphicOpacity=opc_vis_sph  GraphicSpecularColor=[0.5 0.5 0.5 1.0]  GraphicAmbientColor=[0.15 0.15 0.15 1.0]  GraphicEmissiveColor=[0.0 0.0 0.0 1.0]  GraphicShininess=75  DoExposeReferenceFrame=on  SerializedFrames=<Frames/>
  W : PMIOPort  Side=Left
  UAf : PMIOPort  Port=2  Side=Right
  UAr : PMIOPort  Port=3  Side=Right
  UAo : PMIOPort  Port=4  Side=Right
  LAf : PMIOPort  Port=5  Side=Right
  LAr : PMIOPort  Port=6  Side=Right
  LAo : PMIOPort  Port=7  Side=Right
  SpB : PMIOPort  Port=8  Side=Right
  SpT : PMIOPort  Port=9  Side=Right
  RdI : PMIOPort  Port=10  Side=Right
  RdO : PMIOPort  Port=11  Side=Right
  WhC : PMIOPort  Port=12  Side=Right
  connections:
  Graphic Spring Top/RConn1 -- SpT/RConn1 -- Transform Spring Top/RConn1 -- Vis HP Spring Top/RConn1
  Transform UA Outboard/LConn1 -- Transform UA InboardR/LConn1 -- W/RConn1 -- Transform Wheel Center/LConn1 -- Transform Rod Outboard/LConn1 -- Transform Rod Inboard/LConn1 -- Transform Spring Top/LConn1 -- Transform Spring Bottom/LConn1 -- Transform UA InboardF/LConn1 -- Transform LA Outboard/LConn1 -- Transform LA InboardR/LConn1 -- Transform LA InboardF/LConn1
  Transform UA Outboard/RConn1 -- UAo/RConn1 -- Vis HP UA Outboard/RConn1 -- Graphic UA Outboard/RConn1
  Vis HP Spring Bottom/RConn1 -- SpB/RConn1 -- Transform Spring Bottom/RConn1 -- Graphic Spring Bottom/RConn1
  Vis HP LA Outboard/RConn1 -- LAo/RConn1 -- Transform LA Outboard/RConn1 -- Graphic LA Outboard/RConn1
  Graphic Rod Outboard/RConn1 -- RdO/RConn1 -- Transform Rod Outboard/RConn1 -- Vis HP Rod Outboard/RConn1
  Graphic Wheel Center/RConn1 -- WhC/RConn1 -- Transform Wheel Center/RConn1 -- Vis HP Wheel Center/RConn1
  Transform UA InboardF/RConn1 -- UAf/RConn1 -- Graphic UA Inboard F/RConn1 -- Vis HP UA Inboard F/RConn1
  Graphic UA Inboard R/RConn1 -- UAr/RConn1 -- Transform UA InboardR/RConn1 -- Vis HP UA Inboard R/RConn1
  Transform LA InboardF/RConn1 -- LAf/RConn1 -- Graphic LA Inboard F/RConn1 -- Vis HP LA Inboard F/RConn1
  Graphic LA Inboard R/RConn1 -- LAr/RConn1 -- Transform LA InboardR/RConn1 -- Vis HP LA Inboard R/RConn1
  Graphic Rod Inboard/RConn1 -- Vis HP Rod Inboard/RConn1 -- RdI/RConn1 -- Transform Rod Inboard/RConn1
